simulink model "sldemo_boiler"  (Simulink 7.6)
settings: Solver=ode45  StartTime=0.0  StopTime=1400  RelTol=1e-3
Description:
  | Bang-Bang Control Using Temporal Logic
  | 
  | This demonstration shows how to use Stateflow(R) to model a bang-bang temperature
  | control system for a boiler. The boiler dynamics are modeled in Simulink(R).
  | 
  | The Bang-Bang Controller Stateflow chart shows how to use functions and Subcharts
  | within Stateflow.
settings Model: Creator=The MathWorks Inc.  CovMetricSettings=dcmtr  ExtModeTrigMode=oneshot  ExtModeArmWhenConnect=off  ExtModeAutoUpdateStatusClock=off
settings DataIOCC: LimitDataPoints=off  SaveOutput=off  SaveTime=off  SignalLoggingName=sigsOut
settings OptimizationCC: BlockReduction=off  BooleanDataType=off  InitFltsAndDblsToZero=on  OptimizeModelRefInitCode=on  LifeSpan=1
settings DebuggingCC: SaveWithParameterizedLinksMsg=none  SignalResolutionControl=TryResolveAllWithWarning  SolverPrmCheckMsg=none  MultiTaskDSMMsg=warning  MultiTaskCondExecSysMsg=none
settings HardwareCC: ProdHWDeviceType=ASIC/FPGA  TargetUnknown=on
settings SFSimCC: SFSimOverflowDetection=off  SFSimEcho=off  SimParseCustomCode=off
settings RTWCC: SystemTargetFile=ert.tlc  GenCodeOnly=on  TemplateMakefile=ert_default_tmf  GenerateReport=on  RTWVerbose=off  ProcessScript=ert_make_rtw_hook  IncludeHyperlinkInReport=on  LaunchReport=on  IncludeERTFirstTime=on
settings CodeAppCC: IgnoreCustomStorageClasses=off
settings ERTTargetCC: TargetFcnLib=ansi_tfl_tmw.mat  MultiwordLength=2048  GenerateSampleERTMain=on  SupportContinuousTime=on  SupportNonInlinedSFcns=on  InlinedParameterPlacement=NonHierarchical  ERTCustomFileTemplate=example_file_process.tlc  ConvertIfToSwitch=off

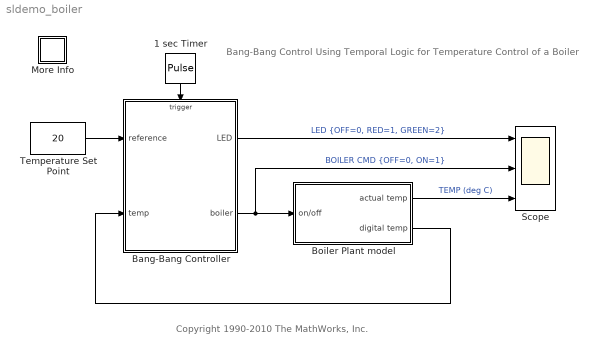
== system sldemo_boiler ==
  note: Bang-Bang Control Using Temporal Logic
      | for Temperature Control of a Boiler
  note: Copyright 1990-2010 The MathWorks, Inc.
  1 sec Timer : DiscretePulseGenerator  Amplitude=int8(1)
  Bang-Bang Controller : Stateflow chart  TreatAsAtomicUnit=on
  Boiler Plant model : Subsystem
  More Info : Subsystem
      settings: OpenFcn=showdemo('sldemo_boiler')
      mask Display: disp('?')
  Scope : Scope  NumInputPorts=3
      settings: YMin=0~0~15  YMax=2~1~24
  Temperature Set Point : Constant  Value=20  OutDataTypeStr=Inherit: Inherit via back propagation
  wires:
  1 sec Timer/1 -> Bang-Bang Controller/Trigger
  Bang-Bang Controller/2(boiler) -> Scope/2, Boiler Plant model/1(on/off)  "BOILER CMD {OFF=0, ON=1}"
  Temperature Set Point/1 -> Bang-Bang Controller/1(reference)
  Boiler Plant model/2(digital temp) -> Bang-Bang Controller/2(temp)
  Boiler Plant model/1(actual temp) -> Scope/3  "TEMP (deg C)"
  Bang-Bang Controller/1(LED) -> Scope/1  "LED {OFF=0, RED=1, GREEN=2}"

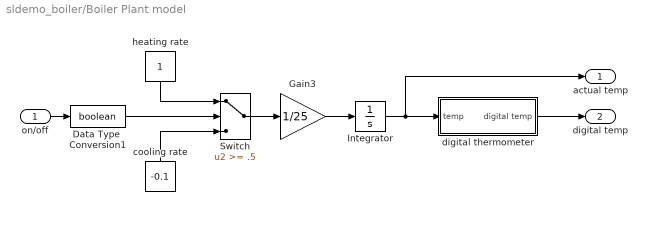
== system sldemo_boiler/Boiler Plant model ==
  on/off : Inport
  Data Type  Conversion1 : DataTypeConversion  OutDataTypeStr=boolean  SaturateOnIntegerOverflow=on  RndMeth=Zero
  Gain3 : Gain  Gain=1/25  SaturateOnIntegerOverflow=on  OutDataTypeStr=Inherit: Same as input  ParamDataTypeStr=Inherit: Same as input
  Integrator : Integrator  InitialCondition=15  ZeroCross=off
  Switch : Switch  Threshold=.5  SaturateOnIntegerOverflow=on  InputSameDT=on
  cooling rate : Constant  Value=-0.1
  digital thermometer : Subsystem
  heating rate : Constant
  actual temp : Outport
  digital temp : Outport  Port=2
  wires:
  Gain3/1 -> Integrator/1
  cooling rate/1 -> Switch/3
  heating rate/1 -> Switch/1
  Switch/1 -> Gain3/1
  on/off/1 -> Data Type  Conversion1/1
  Data Type  Conversion1/1 -> Switch/2
  Integrator/1 -> actual temp/1, digital thermometer/1(temp)
  digital thermometer/1(digital temp) -> digital temp/1

== system sldemo_boiler/More Info ==

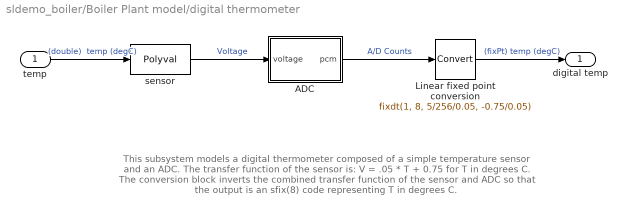
== system sldemo_boiler/Boiler Plant model/digital thermometer ==
  note: This subsystem models a digital thermometer composed of a simple
      | temperature sensor and an ADC.  The transfer function of the sensor is:
      | V = .05 * T + 0.75
      | for T in degrees C.
      |
      | The conversion block inverts the combined transfer function of the sensor
      | and ADC so that the output is an sfix(8) code representing T in degrees C.
  temp : Inport
  ADC : Subsystem
      mask Display: fprintf('ADC\n8-bit\n0-5V');
  Linear fixed point conversion : DataTypeConversion  OutDataTypeStr=fixdt(1, 8, 5/256/0.05, -0.75/0.05)  ConvertRealWorld=Stored Integer (SI)
  sensor : Polyval  Coefs="[ 0.05     0.75 ]"
  digital temp : Outport
  wires:
  sensor/1 -> ADC/1(voltage)  "Voltage"
  ADC/1(pcm) -> Linear fixed point conversion/1  "A/D Counts"
  temp/1 -> sensor/1  "(double)  temp (degC)"
  Linear fixed point conversion/1 -> digital temp/1  "(fixPt) temp (degC)"

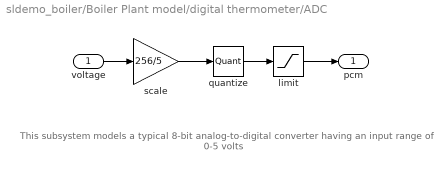
== system sldemo_boiler/Boiler Plant model/digital thermometer/ADC ==
  note: This subsystem models a typical
      | 8-bit analog-to-digital converter
      | having an input range of 0-5 volts
  voltage : Inport
  limit : Saturate  UpperLimit=255  LowerLimit=0
  quantize : Quantizer  QuantizationInterval=1
  scale : Gain  Gain=256/5  SaturateOnIntegerOverflow=on  OutDataTypeStr=Inherit: Same as input  ParamDataTypeStr=Inherit: Same as input
  pcm : Outport
  wires:
  limit/1 -> pcm/1
  scale/1 -> quantize/1
  quantize/1 -> limit/1
  voltage/1 -> scale/1

== stateflow chart Bang-Bang Controller ==
  state Heater [group]
    state Off
      entry: turn_boiler(OFF)
      on every(5,sec): flash_LED()
    state On
      en: turn_boiler(ON)
      du: flash_LED()
      (history)
      state HIGH
      state NORM
      state b = warm() [function]
        (default) -> (junction 22) : {b = !cold()}
      (default) -> HIGH
      HIGH -> NORM : [warm()]
    (default) -> Off
    On -> Off : after(20,sec)
    Off -> On : after(40,sec)
        | [cold()]
    NORM -> Off : [Heater.On.warm()]
  state flash_LED() [function]
    (junction 18) -> (junction 12) [order 2] : {LED=OFF}
    (default) -> (junction 18)
    (junction 18) -> (junction 19) [order 1] : [LED==OFF]
    (junction 19) -> (junction 23) : {LED=color}
  state turn_boiler(mode) [function]
    (default) -> (junction 13)
    (junction 13) -> (junction 14) [order 1] : [mode==ON]
    (junction 16) -> (junction 15)
    (junction 14) -> (junction 16) : {color=GREEN}
    (junction 13) -> (junction 24) [order 2] : {color=RED}
    (junction 15) -> (junction 17) : {LED=color;
        |  boiler=mode}
    (junction 24) -> (junction 15)
  state b = cold() [function]
    (default) -> (junction 20) : { b = temp<=reference}
  data: mode function_input int8; b function_output boolean; b function_output boolean; LED output int8; boiler output int8; color local int8; reference input fixdt(1,8,1,-15); GREEN constant int8 =2; OFF constant int8; ON constant int8 =1; RED constant int8 =1; temp input fixdt(1,8,0.390625,-15)
  events: sec input RISING_EDGE_EVENT
